simulink model "DR"  (R2026a)
settings: Solver=VariableStepAuto  StopTime=168
settings Model: Creator=swastikkumar  LastModifiedBy=swastikkumar

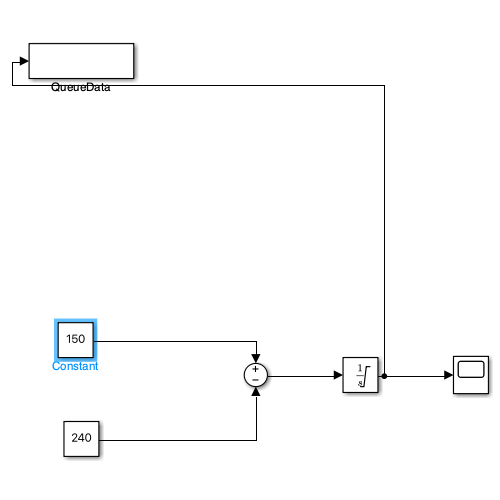
[thumbnail: Simulink's stored preview of the top-level diagram]
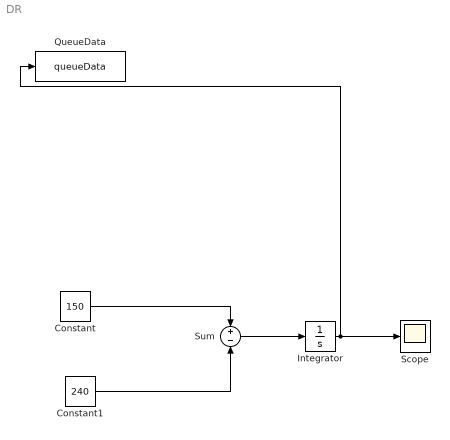
== system DR ==
  Constant : Constant  Value=150
  Constant1 : Constant  Value=240
  Integrator : Integrator  LimitOutput=on  LowerSaturationLimit=0
  QueueData : ToWorkspace  VariableName=queueData  SaveFormat=Structure With Time  SampleTime=-1
  Scope : Scope
  Sum : Sum  Inputs=+-
  wires:
  Constant/1 -> Sum/1
  Constant1/1 -> Sum/2
  Sum/1 -> Integrator/1
  Integrator/1 -> Scope/1, QueueData/1
